simulink model "festo_proiect"  (R2022b)
settings: Solver=ode45  StartTime=0.0  StopTime=1500  RelTol=1e-3
undefined symbols (not defined in the file): A, C, dqi, hinitial, Hr, Hr1, Hr2, k, k1, k2, k3, k_comp, keta, qinitial, ua
libraries: slpidlib x7
(part 2 of 2)

== system festo_proiect/model5/Motor ==
  um : Inport
  im : Inport  Port=2
  Add : Sum  Inputs=+-
  Rm : Gain  Gain=3
  km*n : Outport
  wires:
  Add/1 -> km*n/1
  Rm/1 -> Add/2
  im/1 -> Rm/1
  um/1 -> Add/1

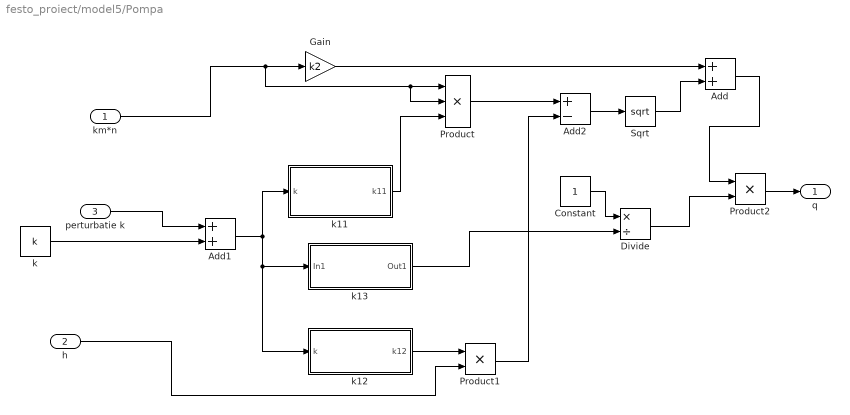
== system festo_proiect/model5/Pompa ==
  km*n : Inport
  h : Inport  Port=2
  perturbatie k : Inport  Port=3
  Add : Sum
  Add1 : Sum
  Add2 : Sum  Inputs=+-
  Constant : Constant
  Divide : Product  Inputs=*/
  Gain : Gain  Gain=k2
  Product : Product  Inputs=3
  Product1 : Product
  Product2 : Product
  Sqrt : Sqrt
  k : Constant  Value=k
  k11 : Subsystem
  k12 : Subsystem
  k13 : Subsystem
  q : Outport
  wires:
  Product2/1 -> q/1
  Divide/1 -> Product2/2
  Constant/1 -> Divide/1
  k13/1(Out1) -> Divide/2
  Add/1 -> Product2/1
  Sqrt/1 -> Add/2
  Add2/1 -> Sqrt/1
  Product1/1 -> Add2/2
  k12/1(k12) -> Product1/1
  h/1 -> Product1/2
  Product/1 -> Add2/1
  Gain/1 -> Add/1
  k11/1(k11) -> Product/3
  Add1/1 -> k13/1(In1), k12/1(k), k11/1(k)
  k/1 -> Add1/2
  perturbatie k/1 -> Add1/1
  km*n/1 -> Gain/1, Product/1, Product/2

== system festo_proiect/model5/Randament pompa ==
  q : Inport
  um : Inport  Port=2
  Gain : Gain  Gain=keta
  Product : Product
  eta : Outport
  wires:
  Product/1 -> eta/1
  Gain/1 -> Product/2
  q/1 -> Product/1
  um/1 -> Gain/1

== system festo_proiect/model5/Rezervor ==
  q : Inport
  Constant : Constant  Value=C
  Gain : Gain  Gain=1/A
  Integrator : Integrator  InitialCondition=hinitial
  Product : Product
  Product1 : Product
  Scope : Scope
  Sqrt : Sqrt
  Sum : Sum  Inputs=|+-
  Sum1 : Sum  Inputs=|++
  step : Step  Commented=on  Time=300  After=2  SampleTime=0
  h : Outport
  disturbance_out : Outport  Port=2
  wires:
  Product1/1 -> disturbance_out/1
  Sum1/1 -> Product/2
  Constant/1 -> Sum1/1
  step/1 -> Product1/2, Sum1/2
  Product/1 -> Scope/1, Sum/2  "qe"
  Sqrt/1 -> Product/1, Product1/1
  Integrator/1 -> h/1, Sqrt/1
  Gain/1 -> Integrator/1
  Sum/1 -> Gain/1
  q/1 -> Sum/1

== system festo_proiect/model6/Amplificator ==
  ua : Inport
  Constant : Constant  Value=8.1
  Gain : Gain  Gain=2.2
  Gain1 : Gain  Gain=2.2
  Gain2 : Gain  Gain=5
  Saturation : Saturate  UpperLimit=22  LowerLimit=0
  Sum : Sum  Inputs=|++
  Sum1 : Sum  Inputs=|+-
  Switch : Switch  Threshold=8.1  SaturateOnIntegerOverflow=off  InputSameDT=off
  um : Outport
  wires:
  Gain2/1 -> Sum/2
  ua/1 -> Switch/2, Gain/1, Sum1/1, Gain1/1
  Gain1/1 -> Sum/1
  Constant/1 -> Sum1/2
  Sum1/1 -> Gain2/1
  Switch/1 -> Saturation/1
  Saturation/1 -> um/1
  Gain/1 -> Switch/3
  Sum/1 -> Switch/1

== system festo_proiect/model6/Curent rotoric ==
  q : Inport
  eta : Inport  Port=2
  h : Inport  Port=3
  um : Inport  Port=4
  "  " : Constant  Value=0.001
  Add : Sum  Inputs=|++
  Add1 : Sum  Inputs=|++
  Divide : Product  Inputs=**/
  Gain : Gain  Gain=2
  Gain1 : Gain  Gain=k
  Gain2 : Gain  Gain=1e4
  Product : Product
  Product1 : Product
  im : Outport
  wires:
  h/1 -> Gain/1
  q/1 -> Divide/2, Gain1/1, Product/2
  Gain/1 -> Add/1
  Product/1 -> Add/2
  um/1 -> Product1/2
  "  "/1 -> Add1/1
  Product1/1 -> Add1/2
  Add/1 -> Divide/1
  Add1/1 -> Divide/3
  Divide/1 -> im/1
  eta/1 -> Gain2/1
  Gain2/1 -> Product1/1
  Gain1/1 -> Product/1

== system festo_proiect/model6/Filtru ==
  q : Inport
  Integrator : Integrator  InitialCondition=qinitial
  Sum : Sum  Inputs=|+-
  q_f : Outport
  wires:
  q/1 -> Sum/1
  Sum/1 -> Integrator/1
  Integrator/1 -> Sum/2, q_f/1

== system festo_proiect/model6/Motor ==
  um : Inport
  im : Inport  Port=2
  Add : Sum  Inputs=+-
  Rm : Gain  Gain=3
  km*n : Outport
  wires:
  um/1 -> Add/1
  im/1 -> Rm/1
  Rm/1 -> Add/2
  Add/1 -> km*n/1

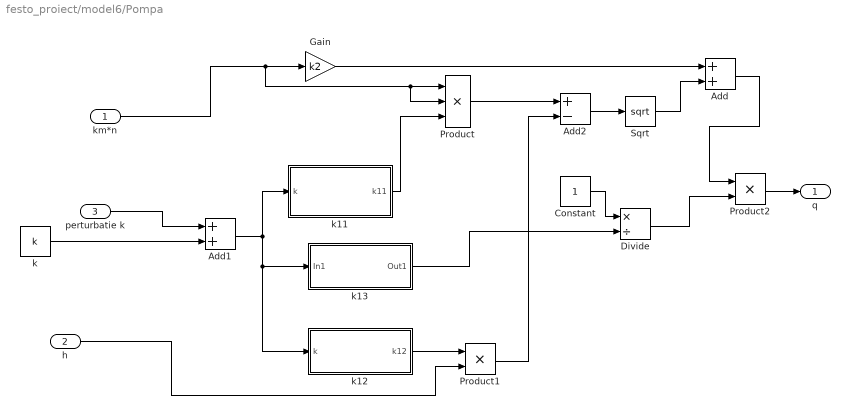
== system festo_proiect/model6/Pompa ==
  km*n : Inport
  h : Inport  Port=2
  perturbatie k : Inport  Port=3
  Add : Sum
  Add1 : Sum
  Add2 : Sum  Inputs=+-
  Constant : Constant
  Divide : Product  Inputs=*/
  Gain : Gain  Gain=k2
  Product : Product  Inputs=3
  Product1 : Product
  Product2 : Product
  Sqrt : Sqrt
  k : Constant  Value=k
  k11 : Subsystem
  k12 : Subsystem
  k13 : Subsystem
  q : Outport
  wires:
  km*n/1 -> Product/2, Product/1, Gain/1
  perturbatie k/1 -> Add1/1
  k/1 -> Add1/2
  Add1/1 -> k11/1(k), k12/1(k), k13/1(In1)
  k11/1(k11) -> Product/3
  Gain/1 -> Add/1
  Product/1 -> Add2/1
  h/1 -> Product1/2
  k12/1(k12) -> Product1/1
  Product1/1 -> Add2/2
  Add2/1 -> Sqrt/1
  Sqrt/1 -> Add/2
  Add/1 -> Product2/1
  k13/1(Out1) -> Divide/2
  Constant/1 -> Divide/1
  Divide/1 -> Product2/2
  Product2/1 -> q/1

== system festo_proiect/model6/Randament pompa ==
  q : Inport
  um : Inport  Port=2
  Gain : Gain  Gain=keta
  Product : Product
  eta : Outport
  wires:
  um/1 -> Gain/1
  q/1 -> Product/1
  Gain/1 -> Product/2
  Product/1 -> eta/1

== system festo_proiect/model6/Rezervor ==
  q : Inport
  Constant : Constant  Value=C
  Gain : Gain  Gain=1/A
  Integrator : Integrator  InitialCondition=hinitial
  Product : Product
  Product1 : Product
  Scope : Scope
  Sqrt : Sqrt
  Sum : Sum  Inputs=|+-
  Sum1 : Sum  Inputs=|++
  step : Step  Time=300  After=2  SampleTime=0
  h : Outport
  disturbance_out : Outport  Port=2
  wires:
  q/1 -> Sum/1
  Sum/1 -> Gain/1
  Gain/1 -> Integrator/1
  Integrator/1 -> Sqrt/1, h/1
  Sqrt/1 -> Product1/1, Product/1
  Product/1 -> Sum/2, Scope/1  "qe"
  step/1 -> Sum1/2, Product1/2
  Constant/1 -> Sum1/1
  Sum1/1 -> Product/2
  Product1/1 -> disturbance_out/1

== system festo_proiect/model/Pompa/k11 ==
  k : Inport
  Add : Sum
  Add1 : Sum  Inputs=+-
  Constant : Constant  Value=k2^2
  Constant1 : Constant  Value=k3
  Gain : Gain  Gain=k1
  Gain1 : Gain  Gain=4
  k11 : Outport
  wires:
  k/1 -> Add1/1
  Constant/1 -> Add/1
  Constant1/1 -> Add1/2
  Add1/1 -> Gain1/1
  Gain1/1 -> Gain/1
  Add/1 -> k11/1
  Gain/1 -> Add/2

== system festo_proiect/model/Pompa/k12 ==
  k : Inport
  Add : Sum  Inputs=+-
  Gain : Gain  Gain=8
  k3 : Constant  Value=k3
  k12 : Outport
  wires:
  Gain/1 -> k12/1
  k/1 -> Add/1
  k3/1 -> Add/2
  Add/1 -> Gain/1

== system festo_proiect/model/Pompa/k13 ==
  In1 : Inport
  Add : Sum  Inputs=+-
  Gain : Gain  Gain=2
  k3 : Constant  Value=k3
  Out1 : Outport
  wires:
  Gain/1 -> Out1/1
  In1/1 -> Add/1
  Add/1 -> Gain/1
  k3/1 -> Add/2

== system festo_proiect/model1/Pompa/k11 ==
  k : Inport
  Add : Sum
  Add1 : Sum  Inputs=+-
  Constant : Constant  Value=k2^2
  Constant1 : Constant  Value=k3
  Gain : Gain  Gain=k1
  Gain1 : Gain  Gain=4
  k11 : Outport
  wires:
  Gain/1 -> Add/2
  Add/1 -> k11/1
  Gain1/1 -> Gain/1
  Add1/1 -> Gain1/1
  Constant1/1 -> Add1/2
  Constant/1 -> Add/1
  k/1 -> Add1/1

== system festo_proiect/model1/Pompa/k12 ==
  k : Inport
  Add : Sum  Inputs=+-
  Gain : Gain  Gain=8
  k3 : Constant  Value=k3
  k12 : Outport
  wires:
  Add/1 -> Gain/1
  k3/1 -> Add/2
  k/1 -> Add/1
  Gain/1 -> k12/1

== system festo_proiect/model1/Pompa/k13 ==
  In1 : Inport
  Add : Sum  Inputs=+-
  Gain : Gain  Gain=2
  k3 : Constant  Value=k3
  Out1 : Outport
  wires:
  k3/1 -> Add/2
  Add/1 -> Gain/1
  In1/1 -> Add/1
  Gain/1 -> Out1/1

== system festo_proiect/model2/Pompa/k11 ==
  k : Inport
  Add : Sum
  Add1 : Sum  Inputs=+-
  Constant : Constant  Value=k2^2
  Constant1 : Constant  Value=k3
  Gain : Gain  Gain=k1
  Gain1 : Gain  Gain=4
  k11 : Outport
  wires:
  k/1 -> Add1/1
  Constant/1 -> Add/1
  Constant1/1 -> Add1/2
  Add1/1 -> Gain1/1
  Gain1/1 -> Gain/1
  Add/1 -> k11/1
  Gain/1 -> Add/2

== system festo_proiect/model2/Pompa/k12 ==
  k : Inport
  Add : Sum  Inputs=+-
  Gain : Gain  Gain=8
  k3 : Constant  Value=k3
  k12 : Outport
  wires:
  Gain/1 -> k12/1
  k/1 -> Add/1
  k3/1 -> Add/2
  Add/1 -> Gain/1

== system festo_proiect/model2/Pompa/k13 ==
  In1 : Inport
  Add : Sum  Inputs=+-
  Gain : Gain  Gain=2
  k3 : Constant  Value=k3
  Out1 : Outport
  wires:
  Gain/1 -> Out1/1
  In1/1 -> Add/1
  Add/1 -> Gain/1
  k3/1 -> Add/2

== system festo_proiect/model3/Pompa/k11 ==
  k : Inport
  Add : Sum
  Add1 : Sum  Inputs=+-
  Constant : Constant  Value=k2^2
  Constant1 : Constant  Value=k3
  Gain : Gain  Gain=k1
  Gain1 : Gain  Gain=4
  k11 : Outport
  wires:
  Gain/1 -> Add/2
  Add/1 -> k11/1
  Gain1/1 -> Gain/1
  Add1/1 -> Gain1/1
  Constant1/1 -> Add1/2
  Constant/1 -> Add/1
  k/1 -> Add1/1

== system festo_proiect/model3/Pompa/k12 ==
  k : Inport
  Add : Sum  Inputs=+-
  Gain : Gain  Gain=8
  k3 : Constant  Value=k3
  k12 : Outport
  wires:
  Add/1 -> Gain/1
  k3/1 -> Add/2
  k/1 -> Add/1
  Gain/1 -> k12/1

== system festo_proiect/model3/Pompa/k13 ==
  In1 : Inport
  Add : Sum  Inputs=+-
  Gain : Gain  Gain=2
  k3 : Constant  Value=k3
  Out1 : Outport
  wires:
  k3/1 -> Add/2
  Add/1 -> Gain/1
  In1/1 -> Add/1
  Gain/1 -> Out1/1

== system festo_proiect/model4/Pompa/k11 ==
  k : Inport
  Add : Sum
  Add1 : Sum  Inputs=+-
  Constant : Constant  Value=k2^2
  Constant1 : Constant  Value=k3
  Gain : Gain  Gain=k1
  Gain1 : Gain  Gain=4
  k11 : Outport
  wires:
  k/1 -> Add1/1
  Constant/1 -> Add/1
  Constant1/1 -> Add1/2
  Add1/1 -> Gain1/1
  Gain1/1 -> Gain/1
  Add/1 -> k11/1
  Gain/1 -> Add/2

== system festo_proiect/model4/Pompa/k12 ==
  k : Inport
  Add : Sum  Inputs=+-
  Gain : Gain  Gain=8
  k3 : Constant  Value=k3
  k12 : Outport
  wires:
  Gain/1 -> k12/1
  k/1 -> Add/1
  k3/1 -> Add/2
  Add/1 -> Gain/1

== system festo_proiect/model4/Pompa/k13 ==
  In1 : Inport
  Add : Sum  Inputs=+-
  Gain : Gain  Gain=2
  k3 : Constant  Value=k3
  Out1 : Outport
  wires:
  Gain/1 -> Out1/1
  In1/1 -> Add/1
  Add/1 -> Gain/1
  k3/1 -> Add/2

== system festo_proiect/model5/Pompa/k11 ==
  k : Inport
  Add : Sum
  Add1 : Sum  Inputs=+-
  Constant : Constant  Value=k2^2
  Constant1 : Constant  Value=k3
  Gain : Gain  Gain=k1
  Gain1 : Gain  Gain=4
  k11 : Outport
  wires:
  Gain/1 -> Add/2
  Add/1 -> k11/1
  Gain1/1 -> Gain/1
  Add1/1 -> Gain1/1
  Constant1/1 -> Add1/2
  Constant/1 -> Add/1
  k/1 -> Add1/1

== system festo_proiect/model5/Pompa/k12 ==
  k : Inport
  Add : Sum  Inputs=+-
  Gain : Gain  Gain=8
  k3 : Constant  Value=k3
  k12 : Outport
  wires:
  Add/1 -> Gain/1
  k3/1 -> Add/2
  k/1 -> Add/1
  Gain/1 -> k12/1

== system festo_proiect/model5/Pompa/k13 ==
  In1 : Inport
  Add : Sum  Inputs=+-
  Gain : Gain  Gain=2
  k3 : Constant  Value=k3
  Out1 : Outport
  wires:
  k3/1 -> Add/2
  Add/1 -> Gain/1
  In1/1 -> Add/1
  Gain/1 -> Out1/1

== system festo_proiect/model6/Pompa/k11 ==
  k : Inport
  Add : Sum
  Add1 : Sum  Inputs=+-
  Constant : Constant  Value=k2^2
  Constant1 : Constant  Value=k3
  Gain : Gain  Gain=k1
  Gain1 : Gain  Gain=4
  k11 : Outport
  wires:
  k/1 -> Add1/1
  Constant/1 -> Add/1
  Constant1/1 -> Add1/2
  Add1/1 -> Gain1/1
  Gain1/1 -> Gain/1
  Add/1 -> k11/1
  Gain/1 -> Add/2

== system festo_proiect/model6/Pompa/k12 ==
  k : Inport
  Add : Sum  Inputs=+-
  Gain : Gain  Gain=8
  k3 : Constant  Value=k3
  k12 : Outport
  wires:
  Gain/1 -> k12/1
  k/1 -> Add/1
  k3/1 -> Add/2
  Add/1 -> Gain/1

== system festo_proiect/model6/Pompa/k13 ==
  In1 : Inport
  Add : Sum  Inputs=+-
  Gain : Gain  Gain=2
  k3 : Constant  Value=k3
  Out1 : Outport
  wires:
  Gain/1 -> Out1/1
  In1/1 -> Add/1
  Add/1 -> Gain/1
  k3/1 -> Add/2
